simulink model "testMat"  (R2023b)
settings: Solver=VariableStepAuto  StartTime=0.0  StopTime=10.0  RelTol=1e-3
libraries: matrix_library x1
settings Model: Creator=jtgrasb  LastModifiedBy=jtgrasb

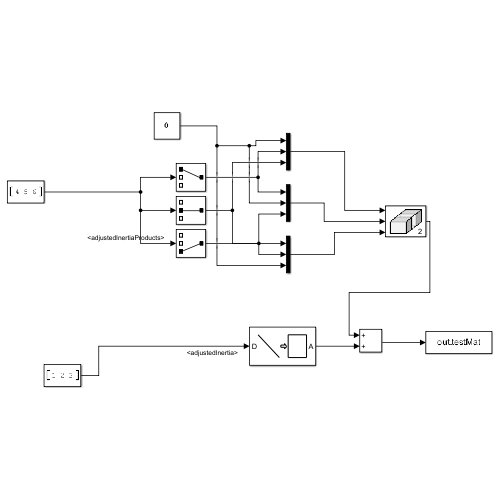
[thumbnail: Simulink's stored preview of the top-level diagram]
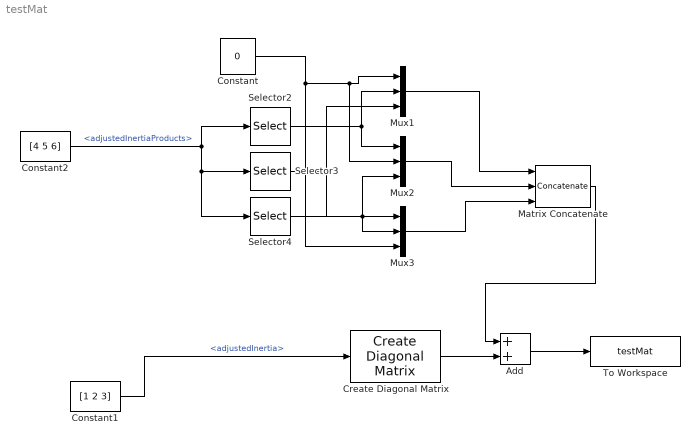
== system testMat ==
  Add : Sum
  Constant : Constant  Value=0
  Constant1 : Constant  Value=[1 2 3]
  Constant2 : Constant  Value=[4 5 6]
  Create Diagonal Matrix : matrix_library/Create Diagonal Matrix
      settings: LibrarySourceBlock=|
      | simulink/Matrix
      | Operations/Create Diagonal
      | Matrix
  Matrix Concatenate : Concatenate  NumInputs=3  Mode=Multidimensional array  ConcatenateDimension=2
  Mux1 : Mux  Inputs=3
  Mux2 : Mux  Inputs=3
  Mux3 : Mux  Inputs=3
  Selector2 : Selector  InputPortWidth=3  IndexOptions=Index vector (dialog)  Indices=1  OutputSizes=1
  Selector3 : Selector  InputPortWidth=3  IndexOptions=Index vector (dialog)  Indices=2  OutputSizes=1
  Selector4 : Selector  InputPortWidth=3  IndexOptions=Index vector (dialog)  Indices=3  OutputSizes=1
  To Workspace : ToWorkspace  VariableName=testMat  SaveFormat=Timeseries  SampleTime=-1
  wires:
  Add/1 -> To Workspace/1
  Matrix Concatenate/1 -> Add/1
  Constant2/1 -> Selector4/1, Selector3/1, Selector2/1  "<adjustedInertiaProducts>"
  Mux3/1 -> Matrix Concatenate/3
  Mux2/1 -> Matrix Concatenate/2
  Mux1/1 -> Matrix Concatenate/1
  Selector2/1 -> Mux2/1, Mux1/2
  Create Diagonal Matrix/1 -> Add/2
  Selector4/1 -> Mux3/2, Mux2/3
  Constant/1 -> Mux3/3, Mux1/1, Mux2/2
  Selector3/1 -> Mux3/1, Mux1/3
  Constant1/1 -> Create Diagonal Matrix/1  "<adjustedInertia>"
